simulink subsystem "contactor_module"  (R2021a)
settings: Solver=VariableStepAuto  StartTime=0.0  StopTime=10.0  RelTol=1e-3
libraries: fl_lib x19, nesl_utility x13
settings Model: Creator=miche  LastModifiedBy=miche

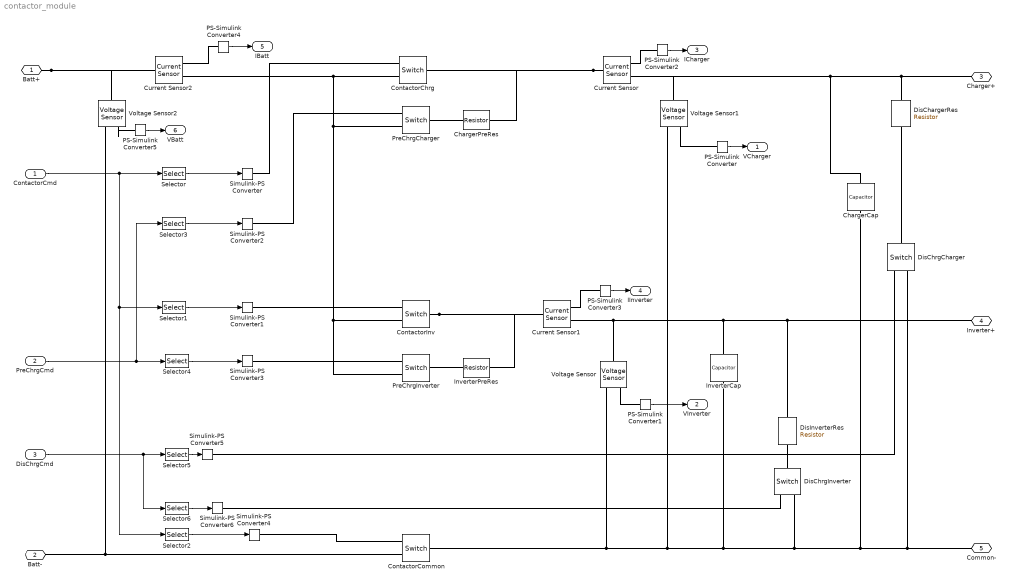
== system contactor_module ==
  ContactorCmd : Inport
  PreChrgCmd : Inport  Port=2
  DisChrgCmd : Inport  Port=3
  ChargerCap : fl_lib/Electrical/Electrical Elements/Capacitor  c=5e-3 F  r=1e-6 Ohm  g=0 1/Ohm  i_specify=off  i_priority=None  i=0 A  i_nominal_specify=off  i_nominal_unit=A  i_nominal_value=1  v_specify=off  v_priority=None  v=0 V  v_nominal_specify=off  v_nominal_unit=V  v_nominal_value=1  vc_specify=off  vc_priority=High  vc=0 V  vc_nominal_specify=off  vc_nominal_unit=V  vc_nominal_value=1
  ChargerPreRes : fl_lib/Electrical/Electrical Elements/Resistor  R=1000 Ohm  i_specify=off  i_priority=None  i=0 A  i_nominal_specify=off  i_nominal_unit=A  i_nominal_value=1  v_specify=off  v_priority=None  v=0 V  v_nominal_specify=off  v_nominal_unit=V  v_nominal_value=1
  ContactorChrg : fl_lib/Electrical/Electrical Elements/Switch  R_closed=0.01 Ohm  G_open=1e-8 1/Ohm  Threshold=0.5  i_specify=off  i_priority=None  i=0 A  i_nominal_specify=off  i_nominal_unit=A  i_nominal_value=1  v_specify=off  v_priority=None  v=0 V  v_nominal_specify=off  v_nominal_unit=V  v_nominal_value=1
  ContactorCommon : fl_lib/Electrical/Electrical Elements/Switch  R_closed=0.01 Ohm  G_open=1e-8 1/Ohm  Threshold=0.5  i_specify=off  i_priority=None  i=0 A  i_nominal_specify=off  i_nominal_unit=A  i_nominal_value=1  v_specify=off  v_priority=None  v=0 V  v_nominal_specify=off  v_nominal_unit=V  v_nominal_value=1
  ContactorInv : fl_lib/Electrical/Electrical Elements/Switch  R_closed=0.01 Ohm  G_open=1e-8 1/Ohm  Threshold=0.5  i_specify=off  i_priority=None  i=0 A  i_nominal_specify=off  i_nominal_unit=A  i_nominal_value=1  v_specify=off  v_priority=None  v=0 V  v_nominal_specify=off  v_nominal_unit=V  v_nominal_value=1
  Current Sensor : fl_lib/Electrical/Electrical Sensors/Current Sensor
  Current Sensor1 : fl_lib/Electrical/Electrical Sensors/Current Sensor
  Current Sensor2 : fl_lib/Electrical/Electrical Sensors/Current Sensor
  DisChargerRes : fl_lib/Electrical/Electrical Elements/Resistor  R=10000 Ohm  i_specify=off  i_priority=None  i=0 A  i_nominal_specify=off  i_nominal_unit=A  i_nominal_value=1  v_specify=off  v_priority=None  v=0 V  v_nominal_specify=off  v_nominal_unit=V  v_nominal_value=1
  DisChrgCharger : fl_lib/Electrical/Electrical Elements/Switch  R_closed=0.01 Ohm  G_open=1e-8 1/Ohm  Threshold=0.5  i_specify=off  i_priority=None  i=0 A  i_nominal_specify=off  i_nominal_unit=A  i_nominal_value=1  v_specify=off  v_priority=None  v=0 V  v_nominal_specify=off  v_nominal_unit=V  v_nominal_value=1
  DisChrgInverter : fl_lib/Electrical/Electrical Elements/Switch  R_closed=0.01 Ohm  G_open=1e-8 1/Ohm  Threshold=0.5  i_specify=off  i_priority=None  i=0 A  i_nominal_specify=off  i_nominal_unit=A  i_nominal_value=1  v_specify=off  v_priority=None  v=0 V  v_nominal_specify=off  v_nominal_unit=V  v_nominal_value=1
  DisInverterRes : fl_lib/Electrical/Electrical Elements/Resistor  R=10000 Ohm  i_specify=off  i_priority=None  i=0 A  i_nominal_specify=off  i_nominal_unit=A  i_nominal_value=1  v_specify=off  v_priority=None  v=0 V  v_nominal_specify=off  v_nominal_unit=V  v_nominal_value=1
  InverterCap : fl_lib/Electrical/Electrical Elements/Capacitor  c=2.5e-3 F  r=1e-6 Ohm  g=0 1/Ohm  i_specify=off  i_priority=None  i=0 A  i_nominal_specify=off  i_nominal_unit=A  i_nominal_value=1  v_specify=off  v_priority=None  v=0 V  v_nominal_specify=off  v_nominal_unit=V  v_nominal_value=1  vc_specify=off  vc_priority=High  vc=0 V  vc_nominal_specify=off  vc_nominal_unit=V  vc_nominal_value=1
  InverterPreRes : fl_lib/Electrical/Electrical Elements/Resistor  R=1000 Ohm  i_specify=off  i_priority=None  i=0 A  i_nominal_specify=off  i_nominal_unit=A  i_nominal_value=1  v_specify=off  v_priority=None  v=0 V  v_nominal_specify=off  v_nominal_unit=V  v_nominal_value=1
  PS-Simulink Converter{,1..5} (6 alike) : nesl_utility/PS-Simulink Converter  PhysicalDomain=network_engine_domain  SubClassName=ps_output  LeftPortType=input  RightPortType=output  PseudoPeriodic=off  Frequencies=[]  Unit=inherit  AffineConversion=off
      settings: SourceProductBaseCode=PW,SS
  PreChrgCharger : fl_lib/Electrical/Electrical Elements/Switch  R_closed=0.01 Ohm  G_open=1e-8 1/Ohm  Threshold=0.5  i_specify=off  i_priority=None  i=0 A  i_nominal_specify=off  i_nominal_unit=A  i_nominal_value=1  v_specify=off  v_priority=None  v=0 V  v_nominal_specify=off  v_nominal_unit=V  v_nominal_value=1
  PreChrgInverter : fl_lib/Electrical/Electrical Elements/Switch  R_closed=0.01 Ohm  G_open=1e-8 1/Ohm  Threshold=0.5  i_specify=off  i_priority=None  i=0 A  i_nominal_specify=off  i_nominal_unit=A  i_nominal_value=1  v_specify=off  v_priority=None  v=0 V  v_nominal_specify=off  v_nominal_unit=V  v_nominal_value=1
  Selector : Selector  InputPortWidth=3  IndexOptions=Index vector (dialog)  Indices=1  OutputSizes=1
  Selector1 : Selector  InputPortWidth=3  IndexOptions=Index vector (dialog)  Indices=2  OutputSizes=1
  Selector2 : Selector  InputPortWidth=3  IndexOptions=Index vector (dialog)  Indices=3  OutputSizes=1
  Selector3 : Selector  InputPortWidth=2  IndexOptions=Index vector (dialog)  Indices=1  OutputSizes=1
  Selector4 : Selector  InputPortWidth=2  IndexOptions=Index vector (dialog)  Indices=2  OutputSizes=1
  Selector5 : Selector  InputPortWidth=2  IndexOptions=Index vector (dialog)  Indices=1  OutputSizes=1
  Selector6 : Selector  InputPortWidth=2  IndexOptions=Index vector (dialog)  Indices=2  OutputSizes=1
  Simulink-PS Converter{,1..6} (7 alike) : nesl_utility/Simulink-PS Converter  PhysicalDomain=network_engine_domain  SubClassName=ps_input  LeftPortType=input  RightPortType=output  PseudoPeriodic=off  Frequencies=[]  NoiseDistribution=none  NoiseParameters=[]  Unit=1  AffineConversion=off  FilteringAndDerivatives=provide  SimscapeFilterOrder=1  InputFilterTimeConstant=0.001  UdotUserProvided=0
      settings: SourceProductBaseCode=PW,SS
  Voltage Sensor : fl_lib/Electrical/Electrical Sensors/Voltage Sensor
  Voltage Sensor1 : fl_lib/Electrical/Electrical Sensors/Voltage Sensor
  Voltage Sensor2 : fl_lib/Electrical/Electrical Sensors/Voltage Sensor
  Batt+ : PMIOPort  Side=Left
  Batt- : PMIOPort  Port=2  Side=Left
  Charger+ : PMIOPort  Port=3  Side=Right
  Inverter+ : PMIOPort  Port=4  Side=Right
  Common- : PMIOPort  Port=5  Side=Right
  VCharger : Outport
  VInverter : Outport  Port=2
  ICharger : Outport  Port=3
  IInverter : Outport  Port=4
  IBatt : Outport  Port=5
  VBatt : Outport  Port=6
  wires:
  Selector/1 -> Simulink-PS Converter/1
  ContactorCmd/1 -> Selector/1, Selector2/1, Selector1/1
  Selector2/1 -> Simulink-PS Converter4/1
  Selector1/1 -> Simulink-PS Converter1/1
  PS-Simulink Converter/1 -> VCharger/1
  PS-Simulink Converter1/1 -> VInverter/1
  Selector4/1 -> Simulink-PS Converter3/1
  PreChrgCmd/1 -> Selector4/1, Selector3/1
  PS-Simulink Converter2/1 -> ICharger/1
  PS-Simulink Converter3/1 -> IInverter/1
  PS-Simulink Converter4/1 -> IBatt/1
  PS-Simulink Converter5/1 -> VBatt/1
  DisChrgCmd/1 -> Selector5/1, Selector6/1
  Selector6/1 -> Simulink-PS Converter6/1
  Selector5/1 -> Simulink-PS Converter5/1
  Selector3/1 -> Simulink-PS Converter2/1
  connections:
  ChargerCap/LConn1 -- DisChargerRes/LConn1 -- Charger+/RConn1 -- Voltage Sensor1/LConn1 -- Current Sensor/RConn2
  Current Sensor2/RConn2 -- ContactorChrg/RConn2 -- PreChrgCharger/RConn2 -- PreChrgInverter/RConn2 -- ContactorInv/RConn2
  Voltage Sensor1/RConn2 -- ContactorCommon/LConn1 -- Voltage Sensor/RConn2 -- InverterCap/RConn1 -- DisChrgCharger/RConn2 -- Common-/RConn1 -- ChargerCap/RConn1 -- DisChrgInverter/RConn2
  Current Sensor/LConn1 -- ChargerPreRes/RConn1 -- ContactorChrg/LConn1
  Voltage Sensor/LConn1 -- Current Sensor1/RConn2 -- InverterCap/LConn1 -- Inverter+/RConn1 -- DisInverterRes/LConn1
  ContactorCommon/RConn2 -- Batt-/RConn1 -- Voltage Sensor2/RConn2
  ContactorInv/LConn1 -- Current Sensor1/LConn1 -- InverterPreRes/RConn1
  Batt+/RConn1 -- Current Sensor2/LConn1 -- Voltage Sensor2/LConn1
  Voltage Sensor/RConn1 -- PS-Simulink Converter1/LConn1
  Simulink-PS Converter3/RConn1 -- PreChrgInverter/RConn1
  Simulink-PS Converter2/RConn1 -- PreChrgCharger/RConn1
  PreChrgCharger/LConn1 -- ChargerPreRes/LConn1
  Simulink-PS Converter4/RConn1 -- ContactorCommon/RConn1
  Simulink-PS Converter/RConn1 -- ContactorChrg/RConn1
  Simulink-PS Converter1/RConn1 -- ContactorInv/RConn1
  Voltage Sensor1/RConn1 -- PS-Simulink Converter/LConn1
  PreChrgInverter/LConn1 -- InverterPreRes/LConn1
  Current Sensor/RConn1 -- PS-Simulink Converter2/LConn1
  Current Sensor1/RConn1 -- PS-Simulink Converter3/LConn1
  Current Sensor2/RConn1 -- PS-Simulink Converter4/LConn1
  Voltage Sensor2/RConn1 -- PS-Simulink Converter5/LConn1
  DisChrgCharger/LConn1 -- DisChargerRes/RConn1
  Simulink-PS Converter6/RConn1 -- DisChrgInverter/RConn1
  DisChrgInverter/LConn1 -- DisInverterRes/RConn1
  DisChrgCharger/RConn1 -- Simulink-PS Converter5/RConn1
